simulink model "q4"  (R2025a)
settings: Solver=VariableStepAuto  StartTime=0.0  StopTime=900  RelTol=1e-3
settings Model: Creator=dtemu  LastModifiedBy=dtemu

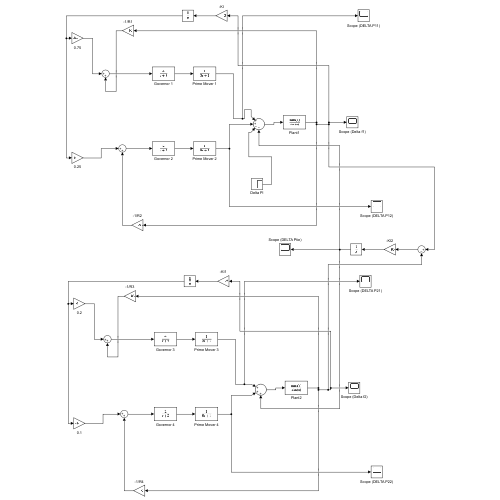
[thumbnail: Simulink's stored preview of the top-level diagram]
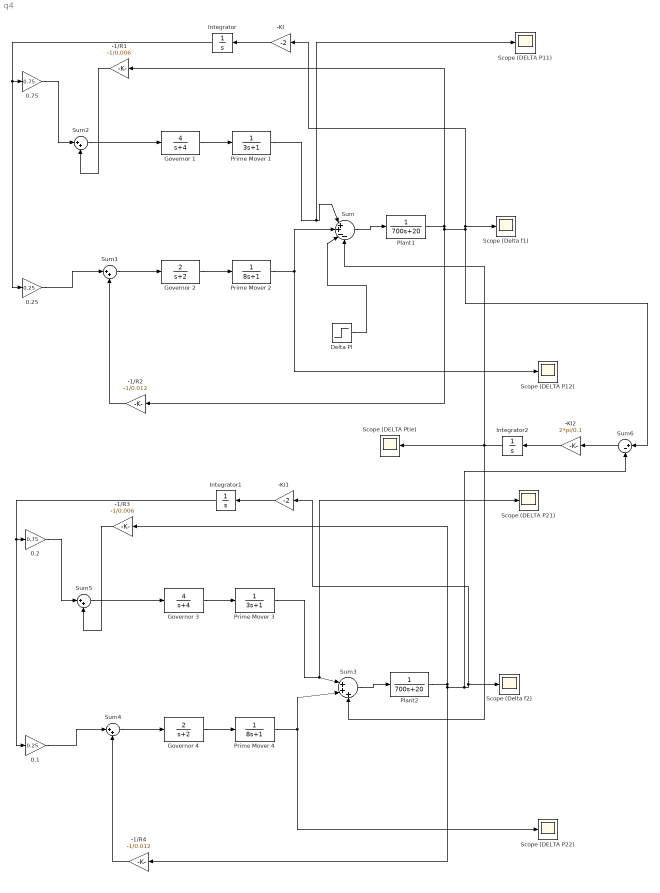
== system q4 ==
  -1/R1 : Gain  Gain=-1/0.006
  -1/R2 : Gain  Gain=-1/0.012
  -1/R3 : Gain  Gain=-1/0.006
  -1/R4 : Gain  Gain=-1/0.012
  -KI : Gain  Gain=-2
  -KI1 : Gain  Gain=-2
  -KI2 : Gain  Gain=2*pi/0.1
  0.1 : Gain  Gain=0.25
  0.2 : Gain  Gain=0.75
  0.25 : Gain  Gain=0.25
  0.75 : Gain  Gain=0.75
  Delta Pl : Step  Time=0  After=100  SampleTime=0
  Governor 1 : TransferFcn  Numerator=[4]  Denominator=[1 4]
  Governor 2 : TransferFcn  Numerator=[2]  Denominator=[1 2]
  Governor 3 : TransferFcn  Numerator=[4]  Denominator=[1 4]
  Governor 4 : TransferFcn  Numerator=[2]  Denominator=[1 2]
  Integrator : Integrator
  Integrator1 : Integrator
  Integrator2 : Integrator
  Plant1 : TransferFcn  Denominator=[700 20]
  Plant2 : TransferFcn  Denominator=[700 20]
  Prime Mover 1 : TransferFcn  Denominator=[3 1]
  Prime Mover 2 : TransferFcn  Denominator=[8 1]
  Prime Mover 3 : TransferFcn  Denominator=[3 1]
  Prime Mover 4 : TransferFcn  Denominator=[8 1]
  Scope (DELTA P11) : Scope
      settings: ActiveDisplayYMinimum=-1  ActiveDisplayYMaximum=1  DataLoggingVariableName=ScopeData2
  Scope (DELTA P12) : Scope
      settings: ActiveDisplayYMinimum=-9.1343623216317518  ActiveDisplayYMaximum=39.336792897922535
  Scope (DELTA P21) : Scope
      settings: ActiveDisplayYMinimum=-1  ActiveDisplayYMaximum=1  DataLoggingVariableName=ScopeData3
  Scope (DELTA P22) : Scope
      settings: ActiveDisplayYMinimum=-9.1343623216317518  ActiveDisplayYMaximum=39.336792897922535  DataLoggingVariableName=ScopeData4
  Scope (DELTA Ptie) : Scope
      settings: ActiveDisplayYMinimum=-81.741204474512259  ActiveDisplayYMaximum=9.0823560527235827  DataLoggingVariableName=ScopeData6
  Scope (Delta f1) : Scope
      settings: ActiveDisplayYMinimum=-0.63110521231046024  ActiveDisplayYMaximum=0.0701228013678289
  Scope (Delta f2) : Scope
      settings: ActiveDisplayYMinimum=-0.63110521231046024  ActiveDisplayYMaximum=0.0701228013678289  DataLoggingVariableName=ScopeData5
  Sum : Sum  Inputs=|++--
  Sum{1..2,4..5} (4 alike) : Sum  Inputs=|++
  Sum3 : Sum  Inputs=|+++
  Sum6 : Sum  Inputs=|+-
  wires:
  -1/R1/1 -> Sum2/2
  Delta Pl/1 -> Sum/3
  -1/R2/1 -> Sum1/2
  Sum1/1 -> Governor 2/1
  -KI/1 -> Integrator/1
  0.75/1 -> Sum2/1
  Governor 2/1 -> Prime Mover 2/1
  Prime Mover 1/1 -> Scope (DELTA P11)/1, Sum/1
  Prime Mover 2/1 -> Scope (DELTA P12)/1, Sum/2
  Sum2/1 -> Governor 1/1
  Plant1/1 -> -KI/1, Scope (Delta f1)/1, Sum6/1, -1/R2/1, -1/R1/1
  0.25/1 -> Sum1/1
  Sum/1 -> Plant1/1
  Integrator/1 -> 0.25/1, 0.75/1
  Governor 1/1 -> Prime Mover 1/1
  -1/R3/1 -> Sum5/2
  -1/R4/1 -> Sum4/2
  Sum4/1 -> Governor 4/1
  -KI1/1 -> Integrator1/1
  0.2/1 -> Sum5/1
  Governor 4/1 -> Prime Mover 4/1
  Prime Mover 3/1 -> Scope (DELTA P21)/1, Sum3/1
  Prime Mover 4/1 -> Scope (DELTA P22)/1, Sum3/2
  Sum5/1 -> Governor 3/1
  Plant2/1 -> Sum6/2, -KI1/1, Scope (Delta f2)/1, -1/R4/1, -1/R3/1
  0.1/1 -> Sum4/1
  Sum3/1 -> Plant2/1
  Integrator1/1 -> 0.1/1, 0.2/1
  Governor 3/1 -> Prime Mover 3/1
  Sum6/1 -> -KI2/1
  -KI2/1 -> Integrator2/1
  Integrator2/1 -> Scope (DELTA Ptie)/1, Sum3/3, Sum/4
